simulink model "hu_flatness"  (R2017b)
settings: Solver=VariableStepAuto  StartTime=0.0  StopTime=102  RelTol=1e-9
libraries: simulink x1
(part 2 of 3)

== matlab function hu_flatness/References ==
  data: t input; references output size=18
function references = fcn(t)
%% specify your references here
g=9.81;
if t>=0 & t<2
tanalpha=-1 ; % slope
if t>=0 & t<1
   [ax_d az_d ax_d_dot az_d_dot ax_d_dot_dot az_d_dot_dot]=nest(t);
    ax_d=ax_d;                   az_d=az_d;
    ax_d_dot=ax_d_dot;           az_d_dot=az_d_dot;
    ax_d_dot_dot=ax_d_dot_dot;   az_d_dot_dot=az_d_dot_dot;
else % t>=1 & t<2
   [ax_d az_d ax_d_dot az_d_dot ax_d_dot_dot az_d_dot_dot]=nest(t-1);
  ax_d=-ax_d;                 az_d=-az_d; % invert the direction for the sake of making end velocity zero
  ax_d_dot=-ax_d_dot;         az_d_dot=-az_d_dot;
  ax_d_dot_dot=-ax_d_dot_dot; az_d_dot_dot=-az_d_dot_dot;   
end  
 r_desired=[0 0 0]'    ;              % reference's positions is not solved here
 r_desired_dot=[0 0 0]'    ;          % reference's velocities is not solved here
 r_desired_dot_dot=[ax_d 0 az_d]'   ;       % reference's accelerations
 r_desired_dot_dot_dot=[ax_d_dot 0 az_d_dot]';      % jerk
 r_desired_dot_dot_dot_dot=[ax_d_dot_dot 0 az_d_dot_dot]' ; % snap
 psi_desired=0 ;                      % reference's yaw angle
 psi_desired_dot=0 ;                  % reference's change rate of yaw angle       
 psi_desired_dot_dot=0;
 
elseif t>=2 & t<4
r_desired=[0 0 0]'    ;              % reference's positions is not solved here
r_desired_dot=[0 0 0]'    ;          % reference's velocities is not solved here
r_desired_dot_dot=[0 0 0]'   ;       % reference's accelerations
r_desired_dot_dot_dot=[0 0 0]';      % jerk
r_desired_dot_dot_dot_dot=[0 0 0]' ; % snap
if t>=2 & t<3
psi_desired=pi/4*(t-2)^2 ;                      % reference's yaw angle
psi_desired_dot=pi/2*(t-2);                  % reference's change rate of yaw angle       
psi_desired_dot_dot=pi/2; 
else % t>=3 & t<4
psi_desired=-pi/4*(t-4)^2+pi/2 ;                      % reference's yaw angle
psi_desired_dot=-pi/2*(t-4);                  % reference's change rate of yaw angle       
psi_desired_dot_dot=-pi/2; 
end 

elseif t>=4 & t<6
tanalpha=1/2;
if t>=4 & t<5
   [ax_d az_d ax_d_dot az_d_dot ax_d_dot_dot az_d_dot_dot]=nest(t-4);
    ax_d=-ax_d;                  az_d=-az_d;
    ax_d_dot=-ax_d_dot;          az_d_dot=-az_d_dot;
    ax_d_dot_dot=-ax_d_dot_dot;  az_d_dot_dot=-az_d_dot_dot;
else % t>=5 & t<6
   [ax_d az_d ax_d_dot az_d_dot ax_d_dot_dot az_d_dot_dot]=nest(t-5);
  ax_d=ax_d;                 az_d=az_d; % invert the direction for the sake of making end velocity zero
  ax_d_dot=ax_d_dot;         az_d_dot=az_d_dot;
  ax_d_dot_dot=ax_d_dot_dot; az_d_dot_dot=az_d_dot_dot;   
end  
 r_desired=[0 0 0]'    ;                    % reference's positions is not solved here
 r_desired_dot=[0 0 0]'    ;                % reference's velocities is not solved here
 r_desired_dot_dot=[ax_d 0 az_d]'   ;       % reference's accelerations
 r_desired_dot_dot_dot=[ax_d_dot 0 az_d_dot]';              % jerk
 r_desired_dot_dot_dot_dot=[ax_d_dot_dot 0 az_d_dot_dot]' ; % snap
 psi_desired=pi/2 ;                      % reference's yaw angle
 psi_desired_dot=0 ;                  % reference's change rate of yaw angle       
 psi_desired_dot_dot=0;

elseif t>=6 & t<8
r_desired=[0 0 0]'    ;              % reference's positions is not solved here
r_desired_dot=[0 0 0]'    ;          % reference's velocities is not solved here
r_desired_dot_dot=[0 0 0]'   ;       % reference's accelerations
r_desired_dot_dot_dot=[0 0 0]';      % jerk
r_desired_dot_dot_dot_dot=[0 0 0]' ; % snap
if t>=6 & t<7
psi_desired=pi/2-pi/4*(t-6)^2 ;                      % reference's yaw angle
psi_desired_dot=-pi/2*(t-6);                  % reference's change rate of yaw angle       
psi_desired_dot_dot=-pi/2; 
else % t>=7 & t<8
psi_desired=pi/4*(t-8)^2 ;                      % reference's yaw angle
psi_desired_dot=pi/2*(t-8);                  % reference's change rate of yaw angle       
psi_desired_dot_dot=pi/2; 
end

elseif t>=8 & t<10
tanalpha=-1;
if t>=8 & t<9
   [ax_d az_d ax_d_dot az_d_dot ax_d_dot_dot az_d_dot_dot]=nest(t-8);
    ax_d=ax_d;                        az_d=az_d;
    ax_d_dot=ax_d_dot;           az_d_dot=az_d_dot;
    ax_d_dot_dot=ax_d_dot_dot;   az_d_dot_dot=az_d_dot_dot;
else % t>=9 & t<10
   [ax_d az_d ax_d_dot az_d_dot ax_d_dot_dot az_d_dot_dot]=nest(t-9);
  ax_d=-ax_d;                 az_d=-az_d; % invert the direction for the sake of making end velocity zero
  ax_d_dot=-ax_d_dot;         az_d_dot=-az_d_dot;
  ax_d_dot_dot=-ax_d_dot_dot; az_d_dot_dot=-az_d_dot_dot;   
end  
 r_desired=[0 0 0]'    ;              % reference's positions is not solved here
 r_desired_dot=[0 0 0]'    ;          % reference's velocities is not solved here
 r_desired_dot_dot=[ax_d 0 az_d]'   ;       % reference's accelerations
 r_desired_dot_dot_dot=[ax_d_dot 0 az_d_dot]';      % jerk
 r_desired_dot_dot_dot_dot=[ax_d_dot_dot 0 az_d_dot_dot]' ; % snap
 psi_desired=0 ;                      % reference's yaw angle
 psi_desired_dot=0 ;                  % reference's change rate of yaw angle       
 psi_desired_dot_dot=0;

elseif t>=10 & t<12
r_desired=[0 0 0]'    ;              % reference's positions is not solved here
r_desired_dot=[0 0 0]'    ;          % reference's velocities is not solved here
r_desired_dot_dot=[0 0 0]'   ;       % reference's accelerations
r_desired_dot_dot_dot=[0 0 0]';      % jerk
r_desired_dot_dot_dot_dot=[0 0 0]' ; % snap
if t>=10 & t<11
psi_desired=pi/4*(t-10)^2 ;                      % reference's yaw angle
psi_desired_dot=pi/2*(t-10);                  % reference's change rate of yaw angle       
psi_desired_dot_dot=pi/2; 
else % t>=11 & t<12
psi_desired=-pi/4*(t-12)^2+pi/2 ;                      % reference's yaw angle
psi_desired_dot=-pi/2*(t-12);                  % reference's change rate of yaw angle       
psi_desired_dot_dot=-pi/2; 
end 

elseif t>=12 & t<14
tanalpha=2;
if t>=12 & t<13
   [ax_d az_d ax_d_dot az_d_dot ax_d_dot_dot az_d_dot_dot]=nest(t-12);
    ax_d=-ax_d;                  az_d=-az_d;
    ax_d_dot=-ax_d_dot;          az_d_dot=-az_d_dot;
    ax_d_dot_dot=-ax_d_dot_dot;  az_d_dot_dot=-az_d_dot_dot;
else % t>=13 & t<14
   [ax_d az_d ax_d_dot az_d_dot ax_d_dot_dot az_d_dot_dot]=nest(t-13);
  ax_d=ax_d;                 az_d=az_d; % invert the direction for the sake of making end velocity zero
  ax_d_dot=ax_d_dot;         az_d_dot=az_d_dot;
  ax_d_dot_dot=ax_d_dot_dot; az_d_dot_dot=az_d_dot_dot;   
end  
 r_desired=[0 0 0]'    ;                    % reference's positions is not solved here
 r_desired_dot=[0 0 0]'    ;                % reference's velocities is not solved here
 r_desired_dot_dot=[ax_d 0 az_d]'   ;       % reference's accelerations
 r_desired_dot_dot_dot=[ax_d_dot 0 az_d_dot]';              % jerk
 r_desired_dot_dot_dot_dot=[ax_d_dot_dot 0 az_d_dot_dot]' ; % snap
 psi_desired=pi/2 ;                      % reference's yaw angle
 psi_desired_dot=0 ;                  % reference's change rate of yaw angle       
 psi_desired_dot_dot=0; 
 
elseif t>=14 & t<16
r_desired=[0 0 0]'    ;              % reference's positions is not solved here
r_desired_dot=[0 0 0]'    ;          % reference's velocities is not solved here
r_desired_dot_dot=[0 0 0]'   ;       % reference's accelerations
r_desired_dot_dot_dot=[0 0 0]';      % jerk
r_desired_dot_dot_dot_dot=[0 0 0]' ; % snap
if t>=14 & t<15
psi_desired=pi/2-pi/4*(t-14)^2 ;                      % reference's yaw angle
psi_desired_dot=-pi/2*(t-14);                  % reference's change rate of yaw angle       
psi_desired_dot_dot=-pi/2; 
else % t>=15 & t<16
psi_desired=pi/4*(t-16)^2 ;                      % reference's yaw angle
psi_desired_dot=pi/2*(t-16);                  % reference's change rate of yaw angle       
psi_desired_dot_dot=pi/2; 
end

elseif t>=16 & t<18
tanalpha=5/3;
if t>=16 & t<17
   [ax_d az_d ax_d_dot az_d_dot ax_d_dot_dot az_d_dot_dot]=nest(t-16);
    ax_d=ax_d;                   az_d=az_d;
    ax_d_dot=ax_d_dot;           az_d_dot=az_d_dot;
    ax_d_dot_dot=ax_d_dot_dot;   az_d_dot_dot=az_d_dot_dot;
else % t>=17 & t<18
   [ax_d az_d ax_d_dot az_d_dot ax_d_dot_dot az_d_dot_dot]=nest(t-17);
  ax_d=-ax_d;                 az_d=-az_d; % invert the direction for the sake of making end velocity zero
  ax_d_dot=-ax_d_dot;         az_d_dot=-az_d_dot;
  ax_d_dot_dot=-ax_d_dot_dot; az_d_dot_dot=-az_d_dot_dot;   
end  
 r_desired=[0 0 0]'    ;              % reference's positions is not solved here
 r_desired_dot=[0 0 0]'    ;          % reference's velocities is not solved here
 r_desired_dot_dot=[ax_d 0 az_d]'   ;       % reference's accelerations
 r_desired_dot_dot_dot=[ax_d_dot 0 az_d_dot]';      % jerk
 r_desired_dot_dot_dot_dot=[ax_d_dot_dot 0 az_d_dot_dot]' ; % snap
 psi_desired=0 ;                      % reference's yaw angle
 psi_desired_dot=0 ;                  % reference's change rate of yaw angle       
 psi_desired_dot_dot=0;
 
elseif t>=18 & t<20
r_desired=[0 0 0]'    ;              % reference's positions is not solved here
r_desired_dot=[0 0 0]'    ;          % reference's velocities is not solved here
r_desired_dot_dot=[0 0 0]'   ;       % reference's accelerations
r_desired_dot_dot_dot=[0 0 0]';      % jerk
r_desired_dot_dot_dot_dot=[0 0 0]' ; % snap
if t>=18 & t<19
psi_desired=pi/4*(t-18)^2 ;                      % reference's yaw angle
psi_desired_dot=pi/2*(t-18);                  % reference's change rate of yaw angle       
psi_desired_dot_dot=pi/2; 
else % t>=19 & t<20
psi_desired=-pi/4*(t-20)^2+pi/2 ;                      % reference's yaw angle
psi_desired_dot=-pi/2*(t-20);                  % reference's change rate of yaw angle       
psi_desired_dot_dot=-pi/2; 
end 

elseif t>=20 & t<22
tanalpha=6 ; % slope
if t>=20 & t<21
   [ax_d az_d ax_d_dot az_d_dot ax_d_dot_dot az_d_dot_dot]=nest(t-20);
    ax_d=1/6*ax_d;                   az_d=1/6*az_d;
    ax_d_dot=1/6*ax_d_dot;           az_d_dot=1/6*az_d_dot;
    ax_d_dot_dot=1/6*ax_d_dot_dot;   az_d_dot_dot=1/6*az_d_dot_dot;
else % t>=21 & t<22
   [ax_d az_d ax_d_dot az_d_dot ax_d_dot_dot az_d_dot_dot]=nest(t-21);
  ax_d=-1/6*ax_d;                 az_d=-1/6*az_d; % invert the direction for the sake of making end velocity zero
  ax_d_dot=-1/6*ax_d_dot;         az_d_dot=-1/6*az_d_dot;
  ax_d_dot_dot=-1/6*ax_d_dot_dot; az_d_dot_dot=-1/6*az_d_dot_dot;   
end  
 r_desired=[0 0 0]'    ;              % reference's positions is not solved here
 r_desired_dot=[0 0 0]'    ;          % reference's velocities is not solved here
 r_desired_dot_dot=[ax_d 0 az_d]'   ;       % reference's accelerations
 r_desired_dot_dot_dot=[ax_d_dot 0 az_d_dot]';      % jerk
 r_desired_dot_dot_dot_dot=[ax_d_dot_dot 0 az_d_dot_dot]' ; % snap
 psi_desired=pi/2 ;                      % reference's yaw angle
 psi_desired_dot=0 ;                  % reference's change rate of yaw angle       
 psi_desired_dot_dot=0;

elseif t>=22 & t<24
r_desired=[0 0 0]'    ;              % reference's positions is not solved here
r_desired_dot=[0 0 0]'    ;          % reference's velocities is not solved here
r_desired_dot_dot=[0 0 0]'   ;       % reference's accelerations
r_desired_dot_dot_dot=[0 0 0]';      % jerk
r_desired_dot_dot_dot_dot=[0 0 0]' ; % snap
if t>=22 & t<23
psi_desired=pi/2-pi/4*(t-22)^2 ;                      % reference's yaw angle
psi_desired_dot=-pi/2*(t-22);                  % reference's change rate of yaw angle       
psi_desired_dot_dot=-pi/2; 
else % t>=23 & t<24
psi_desired=pi/4*(t-24)^2 ;                      % reference's yaw angle
psi_desired_dot=pi/2*(t-24);                  % reference's change rate of yaw angle       
psi_desired_dot_dot=pi/2; 
end

elseif t>=24 & t<26
tanalpha=0 ; % slope
if t>=24 & t<25
   [ax_d az_d ax_d_dot az_d_dot ax_d_dot_dot az_d_dot_dot]=nest(t-24);
    ax_d=4/3*ax_d;                   az_d=4/3*az_d;
    ax_d_dot=4/3*ax_d_dot;           az_d_dot=4/3*az_d_dot;
    ax_d_dot_dot=4/3*ax_d_dot_dot;   az_d_dot_dot=4/3*az_d_dot_dot;
else % t>=25 & t<26
   [ax_d az_d ax_d_dot az_d_dot ax_d_dot_dot az_d_dot_dot]=nest(t-25);
  ax_d=-4/3*ax_d;                 az_d=-4/3*az_d; % invert the direction for the sake of making end velocity zero
  ax_d_dot=-4/3*ax_d_dot;         az_d_dot=-4/3*az_d_dot;
  ax_d_dot_dot=-4/3*ax_d_dot_dot; az_d_dot_dot=-4/3*az_d_dot_dot;   
end  
 r_desired=[0 0 0]'    ;              % reference's positions is not solved here
 r_desired_dot=[0 0 0]'    ;          % reference's velocities is not solved here
 r_desired_dot_dot=[ax_d 0 az_d]'   ;       % reference's accelerations
 r_desired_dot_dot_dot=[ax_d_dot 0 az_d_dot]';      % jerk
 r_desired_dot_dot_dot_dot=[ax_d_dot_dot 0 az_d_dot_dot]' ; % snap
 psi_desired=0 ;                      % reference's yaw angle
 psi_desired_dot=0 ;                  % reference's change rate of yaw angle       
 psi_desired_dot_dot=0;
 
elseif t>=26 & t<28
r_desired=[0 0 0]'    ;              % reference's positions is not solved here
r_desired_dot=[0 0 0]'    ;          % reference's velocities is not solved here
r_desired_dot_dot=[0 0 0]'   ;       % reference's accelerations
r_desired_dot_dot_dot=[0 0 0]';      % jerk
r_desired_dot_dot_dot_dot=[0 0 0]' ; % snap
if t>=26 & t<27
psi_desired=pi/4*(t-26)^2 ;                      % reference's yaw angle
psi_desired_dot=pi/2*(t-26);                  % reference's change rate of yaw angle       
psi_desired_dot_dot=pi/2; 
else % t>=27 & t<28
psi_desired=-pi/4*(t-28)^2+pi/2 ;                      % reference's yaw angle
psi_desired_dot=-pi/2*(t-28);                  % reference's change rate of yaw angle       
psi_desired_dot_dot=-pi/2; 
end 

elseif t>=28 & t<30
tanalpha=-2;
if t>=28 & t<29
   [ax_d az_d ax_d_dot az_d_dot ax_d_dot_dot az_d_dot_dot]=nest(t-28);
    ax_d=-214/292*ax_d;                  az_d=-214/292*az_d;
    ax_d_dot=-214/292*ax_d_dot;          az_d_dot=-214/292*az_d_dot;
    ax_d_dot_dot=-214/292*ax_d_dot_dot;  az_d_dot_dot=-214/292*az_d_dot_dot;
else % t>=29 & t<30
   [ax_d az_d ax_d_dot az_d_dot ax_d_dot_dot az_d_dot_dot]=nest(t-29);
  ax_d=214/292*ax_d;                 az_d=214/292*az_d; % invert the direction for the sake of making end velocity zero
  ax_d_dot=214/292*ax_d_dot;         az_d_dot=214/292*az_d_dot;
  ax_d_dot_dot=214/292*ax_d_dot_dot; az_d_dot_dot=214/292*az_d_dot_dot;   
end  
 r_desired=[0 0 0]'    ;                    % reference's positions is not solved here
 r_desired_dot=[0 0 0]'    ;                % reference's velocities is not solved here
 r_desired_dot_dot=[ax_d 0 az_d]'   ;       % reference's accelerations
 r_desired_dot_dot_dot=[ax_d_dot 0 az_d_dot]';              % jerk
 r_desired_dot_dot_dot_dot=[ax_d_dot_dot 0 az_d_dot_dot]' ; % snap
 psi_desired=pi/2 ;                      % reference's yaw angle
 psi_desired_dot=0 ;                  % reference's change rate of yaw angle       
 psi_desired_dot_dot=0;

elseif t>=30 & t<32
r_desired=[0 0 0]'    ;              % reference's positions is not solved here
r_desired_dot=[0 0 0]'    ;          % reference's velocities is not solved here
r_desired_dot_dot=[0 0 0]'   ;       % reference's accelerations
r_desired_dot_dot_dot=[0 0 0]';      % jerk
r_desired_dot_dot_dot_dot=[0 0 0]' ; % snap
if t>=30 & t<31
psi_desired=pi/2-pi/4*(t-30)^2 ;                      % reference's yaw angle
psi_desired_dot=-pi/2*(t-30);                  % reference's change rate of yaw angle       
psi_desired_dot_dot=-pi/2; 
else % t>=31 & t<32
psi_desired=pi/4*(t-32)^2 ;                      % reference's yaw angle
psi_desired_dot=pi/2*(t-32);                  % reference's change rate of yaw angle       
psi_desired_dot_dot=pi/2; 
end

elseif t>=32 & t<34
if t>=32 & t<33
 r_desired=[0 0 0]'    ;              % reference's positions not solved
 r_desired_dot=[0 0 0]'    ;          % reference's velocities not solved
 r_desired_dot_dot=[0 0 -4/5]'   ;       % reference's accelerations
 r_desired_dot_dot_dot=[0 0 0]';      % jerk
 r_desired_dot_dot_dot_dot=[0 0 0]' ; % snap
else % t>=33 & t<34
 r_desired=[0 0 0]'    ;              % reference's positions not solved
 r_desired_dot=[0 0 0]'    ;          % reference's velocities not solved
 r_desired_dot_dot=[0 0 4/5]'   ;       % reference's accelerations
 r_desired_dot_dot_dot=[0 0 0]';      % jerk
 r_desired_dot_dot_dot_dot=[0 0 0]' ; % snap
end
 psi_desired=0 ;                      % reference's yaw angle
 psi_desired_dot=0 ;                  % reference's change rate of yaw angle       
 psi_desired_dot_dot=0;
 
elseif t>=34 & t<36
r_desired=[0 0 0]'    ;              % reference's positions is not solved here
r_desired_dot=[0 0 0]'    ;          % reference's velocities is not solved here
r_desired_dot_dot=[0 0 0]'   ;       % reference's accelerations
r_desired_dot_dot_dot=[0 0 0]';      % jerk
r_desired_dot_dot_dot_dot=[0 0 0]' ; % snap
if t>=34 & t<35
psi_desired=pi/4*(t-34)^2 ;                      % reference's yaw angle
psi_desired_dot=pi/2*(t-34);                  % reference's change rate of yaw angle       
psi_desired_dot_dot=pi/2; 
else % t>=35 & t<36
psi_desired=-pi/4*(t-36)^2+pi/2 ;                      % reference's yaw angle
psi_desired_dot=-pi/2*(t-36);                  % reference's change rate of yaw angle       
psi_desired_dot_dot=-pi/2; 
end 

elseif t>=36 & t<38
tanalpha=0 ; % slope
if t>=36 & t<37
   [ax_d az_d ax_d_dot az_d_dot ax_d_dot_dot az_d_dot_dot]=nest(t-36);
    ax_d=-1/2*ax_d;                   az_d=-1/2*az_d;
    ax_d_dot=-1/2*ax_d_dot;           az_d_dot=-1/2*az_d_dot;
    ax_d_dot_dot=-1/2*ax_d_dot_dot;   az_d_dot_dot=-1/2*az_d_dot_dot;
else % t>=37 & t<38
   [ax_d az_d ax_d_dot az_d_dot ax_d_dot_dot az_d_dot_dot]=nest(t-37);
  ax_d=1/2*ax_d;                 az_d=1/2*az_d; % invert the direction for the sake of making end velocity zero
  ax_d_dot=1/2*ax_d_dot;         az_d_dot=1/2*az_d_dot;
  ax_d_dot_dot=1/2*ax_d_dot_dot; az_d_dot_dot=1/2*az_d_dot_dot;   
end  
 r_desired=[0 0 0]'    ;              % reference's positions is not solved here
 r_desired_dot=[0 0 0]'    ;          % reference's velocities is not solved here
 r_desired_dot_dot=[ax_d 0 az_d]'   ;       % reference's accelerations
 r_desired_dot_dot_dot=[ax_d_dot 0 az_d_dot]';      % jerk
 r_desired_dot_dot_dot_dot=[ax_d_dot_dot 0 az_d_dot_dot]' ; % snap
 psi_desired=pi/2 ;                      % reference's yaw angle
 psi_desired_dot=0 ;                  % reference's change rate of yaw angle       
 psi_desired_dot_dot=0;
 
elseif t>=38 & t<40
r_desired=[0 0 0]'    ;              % reference's positions is not solved here
r_desired_dot=[0 0 0]'    ;          % reference's velocities is not solved here
r_desired_dot_dot=[0 0 0]'   ;       % reference's accelerations
r_desired_dot_dot_dot=[0 0 0]';      % jerk
r_desired_dot_dot_dot_dot=[0 0 0]' ; % snap
if t>=38 & t<39
psi_desired=pi/2-pi/4*(t-38)^2 ;                      % reference's yaw angle
psi_desired_dot=-pi/2*(t-38);                  % reference's change rate of yaw angle       
psi_desired_dot_dot=-pi/2; 
else % t>=39 & t<40
psi_desired=pi/4*(t-40)^2 ;                      % reference's yaw angle
psi_desired_dot=pi/2*(t-40);                  % reference's change rate of yaw angle       
psi_desired_dot_dot=pi/2; 
end

elseif t>=40 & t<42
if t>=40 & t<41
 r_desired=[0 0 0]'    ;              % reference's positions not solved
 r_desired_dot=[0 0 0]'    ;          % reference's velocities not solved
 r_desired_dot_dot=[0 0 -1/2]'   ;       % reference's accelerations
 r_desired_dot_dot_dot=[0 0 0]';      % jerk
 r_desired_dot_dot_dot_dot=[0 0 0]' ; % snap
else % t>=41 & t<42
 r_desired=[0 0 0]'    ;              % reference's positions not solved
 r_desired_dot=[0 0 0]'    ;          % reference's velocities not solved
 r_desired_dot_dot=[0 0 1/2]'   ;       % reference's accelerations
 r_desired_dot_dot_dot=[0 0 0]';      % jerk
 r_desired_dot_dot_dot_dot=[0 0 0]' ; % snap
end
 psi_desired=0 ;                      % reference's yaw angle
 psi_desired_dot=0 ;                  % reference's change rate of yaw angle       
 psi_desired_dot_dot=0;
 
elseif t>=42 & t<44
r_desired=[0 0 0]'    ;              % reference's positions is not solved here
r_desired_dot=[0 0 0]'    ;          % reference's velocities is not solved here
r_desired_dot_dot=[0 0 0]'   ;       % reference's accelerations
r_desired_dot_dot_dot=[0 0 0]';      % jerk
r_desired_dot_dot_dot_dot=[0 0 0]' ; % snap
if t>=42 & t<43
psi_desired=pi/4*(t-42)^2 ;                      % reference's yaw angle
psi_desired_dot=pi/2*(t-42);                  % reference's change rate of yaw angle       
psi_desired_dot_dot=pi/2; 
else % t>=43 & t<44
psi_desired=-pi/4*(t-44)^2+pi/2 ;                      % reference's yaw angle
psi_desired_dot=-pi/2*(t-44);                  % reference's change rate of yaw angle       
psi_desired_dot_dot=-pi/2; 
end 

elseif t>=44 & t<46
if t>=44 & t<45
 r_desired=[0 0 0]'    ;              % reference's positions not solved
 r_desired_dot=[0 0 0]'    ;          % reference's velocities not solved
 r_desired_dot_dot=[0 0 1/2]'   ;       % reference's accelerations
 r_desired_dot_dot_dot=[0 0 0]';      % jerk
 r_desired_dot_dot_dot_dot=[0 0 0]' ; % snap
else % t>=45 & t<46
 r_desired=[0 0 0]'    ;              % reference's positions not solved
 r_desired_dot=[0 0 0]'    ;          % reference's velocities not solved
 r_desired_dot_dot=[0 0 -1/2]'   ;       % reference's accelerations
 r_desired_dot_dot_dot=[0 0 0]';      % jerk
 r_desired_dot_dot_dot_dot=[0 0 0]' ; % snap
end
 psi_desired=pi/2 ;                      % reference's yaw angle
 psi_desired_dot=0 ;                  % reference's change rate of yaw angle       
 psi_desired_dot_dot=0;
 
elseif t>=46 & t<48
r_desired=[0 0 0]'    ;              % reference's positions is not solved here
r_desired_dot=[0 0 0]'    ;          % reference's velocities is not solved here
r_desired_dot_dot=[0 0 0]'   ;       % reference's accelerations
r_desired_dot_dot_dot=[0 0 0]';      % jerk
r_desired_dot_dot_dot_dot=[0 0 0]' ; % snap
if t>=46 & t<47
psi_desired=pi/2-pi/4*(t-46)^2 ;                      % reference's yaw angle
psi_desired_dot=-pi/2*(t-46);                  % reference's change rate of yaw angle       
psi_desired_dot_dot=-pi/2; 
else % t>=47 & t<48
psi_desired=pi/4*(t-48)^2 ;                      % reference's yaw angle
psi_desired_dot=pi/2*(t-48);                  % reference's change rate of yaw angle       
psi_desired_dot_dot=pi/2; 
end

elseif t>=48 & t<50
tanalpha=0 ; % slope
if t>=48 & t<49
   [ax_d az_d ax_d_dot az_d_dot ax_d_dot_dot az_d_dot_dot]=nest(t-48);
    ax_d=ax_d;                   az_d=az_d;
    ax_d_dot=ax_d_dot;           az_d_dot=az_d_dot;
    ax_d_dot_dot=ax_d_dot_dot;   az_d_dot_dot=az_d_dot_dot;
else % t>=49 & t<50
   [ax_d az_d ax_d_dot az_d_dot ax_d_dot_dot az_d_dot_dot]=nest(t-49);
  ax_d=-ax_d;                 az_d=-az_d; % invert the direction for the sake of making end velocity zero
  ax_d_dot=-ax_d_dot;         az_d_dot=-az_d_dot;
  ax_d_dot_dot=-ax_d_dot_dot; az_d_dot_dot=-az_d_dot_dot;   
end  
 r_desired=[0 0 0]'    ;              % reference's positions is not solved here
 r_desired_dot=[0 0 0]'    ;          % reference's velocities is not solved here
 r_desired_dot_dot=[ax_d 0 az_d]'   ;       % reference's accelerations
 r_desired_dot_dot_dot=[ax_d_dot 0 az_d_dot]';      % jerk
 r_desired_dot_dot_dot_dot=[ax_d_dot_dot 0 az_d_dot_dot]' ; % snap
 psi_desired=0 ;                      % reference's yaw angle
 psi_desired_dot=0 ;                  % reference's change rate of yaw angle       
 psi_desired_dot_dot=0;
 
elseif t>=50 & t<52
if t>=50 & t<51
 r_desired=[0 0 0]'    ;              % reference's positions not solved
 r_desired_dot=[0 0 0]'    ;          % reference's velocities not solved
 r_desired_dot_dot=[0 0 -1/2]'   ;       % reference's accelerations
 r_desired_dot_dot_dot=[0 0 0]';      % jerk
 r_desired_dot_dot_dot_dot=[0 0 0]' ; % snap
else % t>=51 & t<52
 r_desired=[0 0 0]'    ;              % reference's positions not solved
 r_desired_dot=[0 0 0]'    ;          % reference's velocities not solved
 r_desired_dot_dot=[0 0 1/2]'   ;       % reference's accelerations
 r_desired_dot_dot_dot=[0 0 0]';      % jerk
 r_desired_dot_dot_dot_dot=[0 0 0]' ; % snap
end
 psi_desired=0 ;                      % reference's yaw angle
 psi_desired_dot=0 ;                  % reference's change rate of yaw angle       
 psi_desired_dot_dot=0;
 
elseif t>=52 & t<54
r_desired=[0 0 0]'    ;              % reference's positions is not solved here
r_desired_dot=[0 0 0]'    ;          % reference's velocities is not solved here
r_desired_dot_dot=[0 0 0]'   ;       % reference's accelerations
r_desired_dot_dot_dot=[0 0 0]';      % jerk
r_desired_dot_dot_dot_dot=[0 0 0]' ; % snap
if t>=52 & t<53
psi_desired=pi/4*(t-52)^2 ;                      % reference's yaw angle
psi_desired_dot=pi/2*(t-52);                  % reference's change rate of yaw angle       
psi_desired_dot_dot=pi/2; 
else % t>=53 & t<54
psi_desired=-pi/4*(t-54)^2+pi/2 ;                      % reference's yaw angle
psi_desired_dot=-pi/2*(t-54);                  % reference's change rate of yaw angle       
psi_desired_dot_dot=-pi/2; 
end 

elseif t>=54 & t<56
tanalpha=0 ; % slope
if t>=54 & t<55
   [ax_d az_d ax_d_dot az_d_dot ax_d_dot_dot az_d_dot_dot]=nest(t-54);
    ax_d=-ax_d;                   az_d=-az_d;
    ax_d_dot=-ax_d_dot;           az_d_dot=-az_d_dot;
    ax_d_dot_dot=-ax_d_dot_dot;   az_d_dot_dot=-az_d_dot_dot;
else % t>=55 & t<56
   [ax_d az_d ax_d_dot az_d_dot ax_d_dot_dot az_d_dot_dot]=nest(t-55);
  ax_d=ax_d;                 az_d=az_d; % invert the direction for the sake of making end velocity zero
  ax_d_dot=ax_d_dot;         az_d_dot=az_d_dot;
  ax_d_dot_dot=ax_d_dot_dot; az_d_dot_dot=az_d_dot_dot;   
end  
 r_desired=[0 0 0]'    ;              % reference's positions is not solved here
 r_desired_dot=[0 0 0]'    ;          % reference's velocities is not solved here
 r_desired_dot_dot=[ax_d 0 az_d]'   ;       % reference's accelerations
 r_desired_dot_dot_dot=[ax_d_dot 0 az_d_dot]';      % jerk
 r_desired_dot_dot_dot_dot=[ax_d_dot_dot 0 az_d_dot_dot]' ; % snap
 psi_desired=pi/2 ;                      % reference's yaw angle
 psi_desired_dot=0 ;                  % reference's change rate of yaw angle       
 psi_desired_dot_dot=0;
 
elseif t>=56 & t<58
r_desired=[0 0 0]'    ;              % reference's positions is not solved here
r_desired_dot=[0 0 0]'    ;          % reference's velocities is not solved here
r_desired_dot_dot=[0 0 0]'   ;       % reference's accelerations
r_desired_dot_dot_dot=[0 0 0]';      % jerk
r_desired_dot_dot_dot_dot=[0 0 0]' ; % snap
if t>=56 & t<57
psi_desired=pi/2-pi/4*(t-56)^2 ;                      % reference's yaw angle
psi_desired_dot=-pi/2*(t-56);                  % reference's change rate of yaw angle       
psi_desired_dot_dot=-pi/2; 
else % t>=57 & t<58
psi_desired=pi/4*(t-58)^2 ;                      % reference's yaw angle
psi_desired_dot=pi/2*(t-58);                  % reference's change rate of yaw angle       
psi_desired_dot_dot=pi/2; 
end

elseif t>=58 & t<60
tanalpha=0 ; % slope
if t>=58 & t<59
   [ax_d az_d ax_d_dot az_d_dot ax_d_dot_dot az_d_dot_dot]=nest(t-58);
    ax_d=ax_d;                   az_d=az_d;
    ax_d_dot=ax_d_dot;           az_d_dot=az_d_dot;
    ax_d_dot_dot=ax_d_dot_dot;   az_d_dot_dot=az_d_dot_dot;
else % t>=59 & t<60
   [ax_d az_d ax_d_dot az_d_dot ax_d_dot_dot az_d_dot_dot]=nest(t-59);
  ax_d=-ax_d;                 az_d=-az_d; % invert the direction for the sake of making end velocity zero
  ax_d_dot=-ax_d_dot;         az_d_dot=-az_d_dot;
  ax_d_dot_dot=-ax_d_dot_dot; az_d_dot_dot=-az_d_dot_dot;   
end  
 r_desired=[0 0 0]'    ;              % reference's positions is not solved here
 r_desired_dot=[0 0 0]'    ;          % reference's velocities is not solved here
 r_desired_dot_dot=[ax_d 0 az_d]'   ;       % reference's accelerations
 r_desired_dot_dot_dot=[ax_d_dot 0 az_d_dot]';      % jerk
 r_desired_dot_dot_dot_dot=[ax_d_dot_dot 0 az_d_dot_dot]' ; % snap
 psi_desired=0 ;                      % reference's yaw angle
 psi_desired_dot=0 ;                  % reference's change rate of yaw angle       
 psi_desired_dot_dot=0;
 
elseif t>=60 & t<62
r_desired=[0 0 0]'    ;              % reference's positions is not solved here
r_desired_dot=[0 0 0]'    ;          % reference's velocities is not solved here
r_desired_dot_dot=[0 0 0]'   ;       % reference's accelerations
r_desired_dot_dot_dot=[0 0 0]';      % jerk
r_desired_dot_dot_dot_dot=[0 0 0]' ; % snap
if t>=60 & t<61
psi_desired=pi/4*(t-60)^2 ;                      % reference's yaw angle
psi_desired_dot=pi/2*(t-60);                  % reference's change rate of yaw angle       
psi_desired_dot_dot=pi/2; 
else % t>=61 & t<62
psi_desired=-pi/4*(t-62)^2+pi/2 ;                      % reference's yaw angle
psi_desired_dot=-pi/2*(t-62);                  % reference's change rate of yaw angle       
psi_desired_dot_dot=-pi/2; 
end 

elseif t>=62 & t<64
tanalpha=10 ; % slope
if t>=62 & t<63
   [ax_d az_d ax_d_dot az_d_dot ax_d_dot_dot az_d_dot_dot]=nest(t-62);
    ax_d=1311/7050*ax_d;                   az_d=1311/7050*az_d;
    ax_d_dot=1311/7050*ax_d_dot;           az_d_dot=1311/7050*az_d_dot;
    ax_d_dot_dot=1311/7050*ax_d_dot_dot;   az_d_dot_dot=1311/7050*az_d_dot_dot;
else % t>=63 & t<64
   [ax_d az_d ax_d_dot az_d_dot ax_d_dot_dot az_d_dot_dot]=nest(t-63);
  ax_d=-1311/7050*ax_d;                 az_d=-1311/7050*az_d; % invert the direction for the sake of making end velocity zero
  ax_d_dot=-1311/7050*ax_d_dot;         az_d_dot=-1311/7050*az_d_dot;
  ax_d_dot_dot=-1311/7050*ax_d_dot_dot; az_d_dot_dot=-1311/7050*az_d_dot_dot;   
end  
 r_desired=[0 0 0]'    ;                    % reference's positions is not solved here
 r_desired_dot=[0 0 0]'    ;                % reference's velocities is not solved here
 r_desired_dot_dot=[ax_d 0 az_d]'   ;       % reference's accelerations
 r_desired_dot_dot_dot=[ax_d_dot 0 az_d_dot]';      % jerk
 r_desired_dot_dot_dot_dot=[ax_d_dot_dot 0 az_d_dot_dot]' ; % snap
 psi_desired=pi/2 ;                      % reference's yaw angle
 psi_desired_dot=0 ;                  % reference's change rate of yaw angle       
 psi_desired_dot_dot=0;
 
elseif t>=64 & t<66
r_desired=[0 0 0]'    ;              % reference's positions is not solved here
r_desired_dot=[0 0 0]'    ;          % reference's velocities is not solved here
r_desired_dot_dot=[0 0 0]'   ;       % reference's accelerations
r_desired_dot_dot_dot=[0 0 0]';      % jerk
r_desired_dot_dot_dot_dot=[0 0 0]' ; % snap
if t>=64 & t<65
psi_desired=pi/2-pi/4*(t-64)^2 ;                      % reference's yaw angle
psi_desired_dot=-pi/2*(t-64);                  % reference's change rate of yaw angle       
psi_desired_dot_dot=-pi/2; 
else % t>=65 & t<66
psi_desired=pi/4*(t-66)^2 ;                      % reference's yaw angle
psi_desired_dot=pi/2*(t-66);                  % reference's change rate of yaw angle       
psi_desired_dot_dot=pi/2; 
end

elseif t>=66 & t<68
if t>=66 & t<67
 r_desired=[0 0 0]'    ;              % reference's positions not solved
 r_desired_dot=[0 0 0]'    ;          % reference's velocities not solved
 r_desired_dot_dot=[0 0 -1.5]'   ;       % reference's accelerations
 r_desired_dot_dot_dot=[0 0 0]';      % jerk
 r_desired_dot_dot_dot_dot=[0 0 0]' ; % snap
else % t>=67 & t<68
 r_desired=[0 0 0]'    ;              % reference's positions not solved
 r_desired_dot=[0 0 0]'    ;          % reference's velocities not solved
 r_desired_dot_dot=[0 0 1.5]'   ;       % reference's accelerations
 r_desired_dot_dot_dot=[0 0 0]';      % jerk
 r_desired_dot_dot_dot_dot=[0 0 0]' ; % snap
end
 psi_desired=0 ;                      % reference's yaw angle
 psi_desired_dot=0 ;                  % reference's change rate of yaw angle       
 psi_desired_dot_dot=0;
 
elseif t>=68 & t<70
r_desired=[0 0 0]'    ;              % reference's positions is not solved here
r_desired_dot=[0 0 0]'    ;          % reference's velocities is not solved here
r_desired_dot_dot=[0 0 0]'   ;       % reference's accelerations
r_desired_dot_dot_dot=[0 0 0]';      % jerk
r_desired_dot_dot_dot_dot=[0 0 0]' ; % snap
if t>=68 & t<69
psi_desired=pi/4*(t-68)^2 ;                      % reference's yaw angle
psi_desired_dot=pi/2*(t-68);                  % reference's change rate of yaw angle       
psi_desired_dot_dot=pi/2; 
else % t>=69 & t<70
psi_desired=-pi/4*(t-70)^2+pi/2 ;                      % reference's yaw angle
psi_desired_dot=-pi/2*(t-70);                  % reference's change rate of yaw angle       
psi_desired_dot_dot=-pi/2; 
end

elseif t>=70 & t<72
if t>=70 & t<71
 r_desired=[0 0 0]'    ;              % reference's positions not solved
 r_desired_dot=[0 0 0]'    ;          % reference's velocities not solved
 r_desired_dot_dot=[0 0 1.5]'   ;       % reference's accelerations
 r_desired_dot_dot_dot=[0 0 0]';      % jerk
 r_desired_dot_dot_dot_dot=[0 0 0]' ; % snap
else % t>=71 & t<72
 r_desired=[0 0 0]'    ;              % reference's positions not solved
 r_desired_dot=[0 0 0]'    ;          % reference's velocities not solved
 r_desired_dot_dot=[0 0 -1.5]'   ;       % reference's accelerations
 r_desired_dot_dot_dot=[0 0 0]';      % jerk
 r_desired_dot_dot_dot_dot=[0 0 0]' ; % snap
end
 psi_desired=pi/2 ;                      % reference's yaw angle
 psi_desired_dot=0 ;                  % reference's change rate of yaw angle       
 psi_desired_dot_dot=0;
 
elseif t>=72 & t<74
r_desired=[0 0 0]'    ;              % reference's positions is not solved here
r_desired_dot=[0 0 0]'    ;          % reference's velocities is not solved here
r_desired_dot_dot=[0 0 0]'   ;       % reference's accelerations
r_desired_dot_dot_dot=[0 0 0]';      % jerk
r_desired_dot_dot_dot_dot=[0 0 0]' ; % snap
if t>=72 & t<73
psi_desired=pi/2-pi/4*(t-72)^2 ;                      % reference's yaw angle
psi_desired_dot=-pi/2*(t-72);                  % reference's change rate of yaw angle       
psi_desired_dot_dot=-pi/2; 
else % t>=73 & t<74
psi_desired=pi/4*(t-74)^2 ;                      % reference's yaw angle
psi_desired_dot=pi/2*(t-74);                  % reference's change rate of yaw angle       
psi_desired_dot_dot=pi/2;    
end

elseif t>=74 & t<76
tanalpha=0 ; % slope
if t>=74 & t<75
   [ax_d az_d ax_d_dot az_d_dot ax_d_dot_dot az_d_dot_dot]=nest(t-74);
    ax_d=ax_d;                   az_d=az_d;
    ax_d_dot=ax_d_dot;           az_d_dot=az_d_dot;
    ax_d_dot_dot=ax_d_dot_dot;   az_d_dot_dot=az_d_dot_dot;
else % t>=75 & t<76
   [ax_d az_d ax_d_dot az_d_dot ax_d_dot_dot az_d_dot_dot]=nest(t-75);
  ax_d=-ax_d;                 az_d=-az_d; % invert the direction for the sake of making end velocity zero
  ax_d_dot=-ax_d_dot;         az_d_dot=-az_d_dot;
  ax_d_dot_dot=-ax_d_dot_dot; az_d_dot_dot=-az_d_dot_dot;   
end  
 r_desired=[0 0 0]'    ;              % reference's positions is not solved here
 r_desired_dot=[0 0 0]'    ;          % reference's velocities is not solved here
 r_desired_dot_dot=[ax_d 0 az_d]'   ;       % reference's accelerations
 r_desired_dot_dot_dot=[ax_d_dot 0 az_d_dot]';      % jerk
 r_desired_dot_dot_dot_dot=[ax_d_dot_dot 0 az_d_dot_dot]' ; % snap
 psi_desired=0 ;                      % reference's yaw angle
 psi_desired_dot=0 ;                  % reference's change rate of yaw angle       
 psi_desired_dot_dot=0;   
 
elseif t>=76 & t<78
if t>=76 & t<77
 r_desired=[0 0 0]'    ;              % reference's positions not solved
 r_desired_dot=[0 0 0]'    ;          % reference's velocities not solved
 r_desired_dot_dot=[0 0 -1.5]'   ;       % reference's accelerations
 r_desired_dot_dot_dot=[0 0 0]';      % jerk
 r_desired_dot_dot_dot_dot=[0 0 0]' ; % snap
else % t>=77 & t<78
 r_desired=[0 0 0]'    ;              % reference's positions not solved
 r_desired_dot=[0 0 0]'    ;          % reference's velocities not solved
 r_desired_dot_dot=[0 0 1.5]'   ;       % reference's accelerations
 r_desired_dot_dot_dot=[0 0 0]';      % jerk
 r_desired_dot_dot_dot_dot=[0 0 0]' ; % snap
end
 psi_desired=0 ;                      % reference's yaw angle
 psi_desired_dot=0 ;                  % reference's change rate of yaw angle       
 psi_desired_dot_dot=0;
 
elseif t>=78 & t<80
tanalpha=0 ; % slope
if t>=78 & t<79
   [ax_d az_d ax_d_dot az_d_dot ax_d_dot_dot az_d_dot_dot]=nest(t-78);
    ax_d=-1/3*ax_d;                   az_d=-1/3*az_d;
    ax_d_dot=-1/3*ax_d_dot;           az_d_dot=-1/3*az_d_dot;
    ax_d_dot_dot=-1/3*ax_d_dot_dot;   az_d_dot_dot=-1/3*az_d_dot_dot;
else % t>=79 & t<80
   [ax_d az_d ax_d_dot az_d_dot ax_d_dot_dot az_d_dot_dot]=nest(t-79);
  ax_d=1/3*ax_d;                 az_d=1/3*az_d; % invert the direction for the sake of making end velocity zero
  ax_d_dot=1/3*ax_d_dot;         az_d_dot=1/3*az_d_dot;
  ax_d_dot_dot=1/3*ax_d_dot_dot; az_d_dot_dot=1/3*az_d_dot_dot;   
end  
 r_desired=[0 0 0]'    ;              % reference's positions is not solved here
 r_desired_dot=[0 0 0]'    ;          % reference's velocities is not solved here
 r_desired_dot_dot=[ax_d 0 az_d]'   ;       % reference's accelerations
 r_desired_dot_dot_dot=[ax_d_dot 0 az_d_dot]';      % jerk
 r_desired_dot_dot_dot_dot=[ax_d_dot_dot 0 az_d_dot_dot]' ; % snap
 psi_desired=0 ;                      % reference's yaw angle
 psi_desired_dot=0 ;                  % reference's change rate of yaw angle       
 psi_desired_dot_dot=0;   
 
elseif t>=80 & t<82
r_desired=[0 0 0]'    ;              % reference's positions is not solved here
r_desired_dot=[0 0 0]'    ;          % reference's velocities is not solved here
r_desired_dot_dot=[0 0 0]'   ;       % reference's accelerations
r_desired_dot_dot_dot=[0 0 0]';      % jerk
r_desired_dot_dot_dot_dot=[0 0 0]' ; % snap
if t>=80 & t<81
psi_desired=pi/4*(t-80)^2 ;                      % reference's yaw angle
psi_desired_dot=pi/2*(t-80);                  % reference's change rate of yaw angle       
psi_desired_dot_dot=pi/2; 
else % t>=81 & t<82
psi_desired=-pi/4*(t-82)^2+pi/2 ;                      % reference's yaw angle
psi_desired_dot=-pi/2*(t-82);                  % reference's change rate of yaw angle       
psi_desired_dot_dot=-pi/2; 
end

elseif t>=82 & t<84
tanalpha=-5 ; % slope
if t>=82 & t<83
   [ax_d az_d ax_d_dot az_d_dot ax_d_dot_dot az_d_dot_dot]=nest(t-82);
    ax_d=-214/258*ax_d;                   az_d=-214/258*az_d;
    ax_d_dot=-214/258*ax_d_dot;           az_d_dot=-214/258*az_d_dot;
    ax_d_dot_dot=-214/258*ax_d_dot_dot;   az_d_dot_dot=-214/258*az_d_dot_dot;
else % t>=83 & t<84
   [ax_d az_d ax_d_dot az_d_dot ax_d_dot_dot az_d_dot_dot]=nest(t-83);
  ax_d=214/258*ax_d;                 az_d=214/258*az_d; % invert the direction for the sake of making end velocity zero
  ax_d_dot=214/258*ax_d_dot;         az_d_dot=214/258*az_d_dot;
  ax_d_dot_dot=214/258*ax_d_dot_dot; az_d_dot_dot=214/258*az_d_dot_dot;   
end  
 r_desired=[0 0 0]'    ;              % reference's positions is not solved here
 r_desired_dot=[0 0 0]'    ;          % reference's velocities is not solved here
 r_desired_dot_dot=[ax_d 0 az_d]'   ;       % reference's accelerations
 r_desired_dot_dot_dot=[ax_d_dot 0 az_d_dot]';      % jerk
 r_desired_dot_dot_dot_dot=[ax_d_dot_dot 0 az_d_dot_dot]' ; % snap
 psi_desired=pi/2 ;                      % reference's yaw angle
 psi_desired_dot=0 ;                  % reference's change rate of yaw angle       
 psi_desired_dot_dot=0; 
 
elseif t>=84 & t<86
r_desired=[0 0 0]'    ;              % reference's positions is not solved here
r_desired_dot=[0 0 0]'    ;          % reference's velocities is not solved here
r_desired_dot_dot=[0 0 0]'   ;       % reference's accelerations
r_desired_dot_dot_dot=[0 0 0]';      % jerk
r_desired_dot_dot_dot_dot=[0 0 0]' ; % snap
if t>=84 & t<85
psi_desired=pi/2-pi/4*(t-84)^2 ;                      % reference's yaw angle
psi_desired_dot=-pi/2*(t-84);                  % reference's change rate of yaw angle       
psi_desired_dot_dot=-pi/2; 
else % t>=85 & t<86
psi_desired=pi/4*(t-86)^2 ;                      % reference's yaw angle
psi_desired_dot=pi/2*(t-86);                  % reference's change rate of yaw angle       
psi_desired_dot_dot=pi/2; 
end

elseif t>=86 & t<88
tanalpha=0 ; % slope
if t>=86 & t<87
   [ax_d az_d ax_d_dot az_d_dot ax_d_dot_dot az_d_dot_dot]=nest(t-86);
    ax_d=ax_d;                   az_d=az_d;
    ax_d_dot=ax_d_dot;           az_d_dot=az_d_dot;
    ax_d_dot_dot=ax_d_dot_dot;   az_d_dot_dot=az_d_dot_dot;
else % t>=87 & t<88
   [ax_d az_d ax_d_dot az_d_dot ax_d_dot_dot az_d_dot_dot]=nest(t-87);
  ax_d=-ax_d;                 az_d=-az_d; % invert the direction for the sake of making end velocity zero
  ax_d_dot=-ax_d_dot;         az_d_dot=-az_d_dot;
  ax_d_dot_dot=-ax_d_dot_dot; az_d_dot_dot=-az_d_dot_dot;   
end  
 r_desired=[0 0 0]'    ;              % reference's positions is not solved here
 r_desired_dot=[0 0 0]'    ;          % reference's velocities is not solved here
 r_desired_dot_dot=[ax_d 0 az_d]'   ;       % reference's accelerations
 r_desired_dot_dot_dot=[ax_d_dot 0 az_d_dot]';      % jerk
 r_desired_dot_dot_dot_dot=[ax_d_dot_dot 0 az_d_dot_dot]' ; % snap
 psi_desired=0 ;                      % reference's yaw angle
 psi_desired_dot=0 ;                  % reference's change rate of yaw angle       
 psi_desired_dot_dot=0; 

elseif t>=88 & t<90
r_desired=[0 0 0]'    ;              % reference's positions is not solved here
r_desired_dot=[0 0 0]'    ;          % reference's velocities is not solved here
r_desired_dot_dot=[0 0 0]'   ;       % reference's accelerations
r_desired_dot_dot_dot=[0 0 0]';      % jerk
r_desired_dot_dot_dot_dot=[0 0 0]' ; % snap
if t>=88 & t<89
psi_desired=pi/4*(t-88)^2 ;                      % reference's yaw angle
psi_desired_dot=pi/2*(t-88);                  % reference's change rate of yaw angle       
psi_desired_dot_dot=pi/2; 
else % t>=89 & t<90
psi_desired=-pi/4*(t-90)^2+pi/2 ;                      % reference's yaw angle
psi_desired_dot=-pi/2*(t-90);                  % reference's change rate of yaw angle       
psi_desired_dot_dot=-pi/2; 
end 

elseif t>=90 & t<92
tanalpha=5/3 ; % slope
if t>=90 & t<91
   [ax_d az_d ax_d_dot az_d_dot ax_d_dot_dot az_d_dot_dot]=nest(t-90);
    ax_d=-321/351*ax_d;                   az_d=-321/351*az_d;
    ax_d_dot=-321/351*ax_d_dot;           az_d_dot=-321/351*az_d_dot;
    ax_d_dot_dot=-321/351*ax_d_dot_dot;   az_d_dot_dot=-321/351*az_d_dot_dot;
else % t>=91 & t<92
   [ax_d az_d ax_d_dot az_d_dot ax_d_dot_dot az_d_dot_dot]=nest(t-91);
  ax_d=321/351*ax_d;                 az_d=321/351*az_d; % invert the direction for the sake of making end velocity zero
  ax_d_dot=321/351*ax_d_dot;         az_d_dot=321/351*az_d_dot;
  ax_d_dot_dot=321/351*ax_d_dot_dot; az_d_dot_dot=321/351*az_d_dot_dot;   
end  
 r_desired=[0 0 0]'    ;              % reference's positions is not solved here
 r_desired_dot=[0 0 0]'    ;          % reference's velocities is not solved here
 r_desired_dot_dot=[ax_d 0 az_d]'   ;       % reference's accelerations
 r_desired_dot_dot_dot=[ax_d_dot 0 az_d_dot]';      % jerk
 r_desired_dot_dot_dot_dot=[ax_d_dot_dot 0 az_d_dot_dot]' ; % snap
 psi_desired=pi/2 ;                      % reference's yaw angle
 psi_desired_dot=0 ;                  % reference's change rate of yaw angle       
 psi_desired_dot_dot=0 ;
 
elseif t>=92 & t<94
r_desired=[0 0 0]'    ;              % reference's positions is not solved here
r_desired_dot=[0 0 0]'    ;          % reference's velocities is not solved here
r_desired_dot_dot=[0 0 0]'   ;       % reference's accelerations
r_desired_dot_dot_dot=[0 0 0]';      % jerk
r_desired_dot_dot_dot_dot=[0 0 0]' ; % snap
if t>=92 & t<93
psi_desired=pi/2-pi/4*(t-92)^2 ;                      % reference's yaw angle
psi_desired_dot=-pi/2*(t-92);                  % reference's change rate of yaw angle       
psi_desired_dot_dot=-pi/2; 
else % t>=93 & t<94
psi_desired=pi/4*(t-94)^2 ;                      % reference's yaw angle
psi_desired_dot=pi/2*(t-94);                  % reference's change rate of yaw angle       
psi_desired_dot_dot=pi/2; 
end

elseif t>=94 & t<96
tanalpha=0 ; % slope
if t>=94 & t<95
   [ax_d az_d ax_d_dot az_d_dot ax_d_dot_dot az_d_dot_dot]=nest(t-94);
    ax_d=ax_d;                   az_d=az_d;
    ax_d_dot=ax_d_dot;           az_d_dot=az_d_dot;
    ax_d_dot_dot=ax_d_dot_dot;   az_d_dot_dot=az_d_dot_dot;
else % t>=95 & t<96
   [ax_d az_d ax_d_dot az_d_dot ax_d_dot_dot az_d_dot_dot]=nest(t-95);
  ax_d=-ax_d;                 az_d=-az_d; % invert the direction for the sake of making end velocity zero
  ax_d_dot=-ax_d_dot;         az_d_dot=-az_d_dot;
  ax_d_dot_dot=-ax_d_dot_dot; az_d_dot_dot=-az_d_dot_dot;   
end  
 r_desired=[0 0 0]'    ;              % reference's positions is not solved here
 r_desired_dot=[0 0 0]'    ;          % reference's velocities is not solved here
 r_desired_dot_dot=[ax_d 0 az_d]'   ;       % reference's accelerations
 r_desired_dot_dot_dot=[ax_d_dot 0 az_d_dot]';      % jerk
 r_desired_dot_dot_dot_dot=[ax_d_dot_dot 0 az_d_dot_dot]' ; % snap
 psi_desired=0 ;                      % reference's yaw angle
 psi_desired_dot=0 ;                  % reference's change rate of yaw angle       
 psi_desired_dot_dot=0; 
 
elseif t>=96 & t<98
r_desired=[0 0 0]'    ;              % reference's positions is not solved here
r_desired_dot=[0 0 0]'    ;          % reference's velocities is not solved here
r_desired_dot_dot=[0 0 0]'   ;       % reference's accelerations
r_desired_dot_dot_dot=[0 0 0]';      % jerk
r_desired_dot_dot_dot_dot=[0 0 0]' ; % snap
if t>=96 & t<97
psi_desired=pi/4*(t-96)^2 ;                      % reference's yaw angle
psi_desired_dot=pi/2*(t-96);                  % reference's change rate of yaw angle       
psi_desired_dot_dot=pi/2; 
else % t>=97 & t<98
psi_desired=-pi/4*(t-98)^2+pi/2 ;                      % reference's yaw angle
psi_desired_dot=-pi/2*(t-98);                  % reference's change rate of yaw angle       
psi_desired_dot_dot=-pi/2; 
end 

elseif t>=98 & t<100
tanalpha=5/3 ; % slope
if t>=98 & t<99
   [ax_d az_d ax_d_dot az_d_dot ax_d_dot_dot az_d_dot_dot]=nest(t-98);
    ax_d=6/7*ax_d;                   az_d=6/7*az_d;
    ax_d_dot=6/7*ax_d_dot;           az_d_dot=6/7*az_d_dot;
    ax_d_dot_dot=6/7*ax_d_dot_dot;   az_d_dot_dot=6/7*az_d_dot_dot;
else % t>=99 & t<100
   [ax_d az_d ax_d_dot az_d_dot ax_d_dot_dot az_d_dot_dot]=nest(t-99);
  ax_d=-6/7*ax_d;                 az_d=-6/7*az_d; % invert the direction for the sake of making end velocity zero
  ax_d_dot=-6/7*ax_d_dot;         az_d_dot=-6/7*az_d_dot;
  ax_d_dot_dot=-6/7*ax_d_dot_dot; az_d_dot_dot=-6/7*az_d_dot_dot;   
end  
 r_desired=[0 0 0]'    ;              % reference's positions is not solved here
 r_desired_dot=[0 0 0]'    ;          % reference's velocities is not solved here
 r_desired_dot_dot=[ax_d 0 az_d]'   ;       % reference's accelerations
 r_desired_dot_dot_dot=[ax_d_dot 0 az_d_dot]';      % jerk
 r_desired_dot_dot_dot_dot=[ax_d_dot_dot 0 az_d_dot_dot]' ; % snap
 psi_desired=pi/2 ;                      % reference's yaw angle
 psi_desired_dot=0 ;                  % reference's change rate of yaw angle       
 psi_desired_dot_dot=0;  
 
else
r_desired=[0 0 0]'    ;              % reference's positions is not solved here
r_desired_dot=[0 0 0]'    ;          % reference's velocities is not solved here
r_desired_dot_dot=[0 0 0]'   ;       % reference's accelerations
r_desired_dot_dot_dot=[0 0 0]';      % jerk
r_desired_dot_dot_dot_dot=[0 0 0]' ; % snap
if t>=100 & t<101
psi_desired=pi/2-pi/4*(t-100)^2 ;                      % reference's yaw angle
psi_desired_dot=-pi/2*(t-100);                  % reference's change rate of yaw angle       
psi_desired_dot_dot=-pi/2; 
else % t>=101 & t<102
psi_desired=pi/4*(t-102)^2 ;                      % reference's yaw angle
psi_desired_dot=pi/2*(t-102);                  % reference's change rate of yaw angle       
psi_desired_dot_dot=pi/2; 
end
end

    
 function   [axn azn axn_dot azn_dot axn_dot_dot azn_dot_dot]=nest(tn)
        if tn>=0 & tn<1/4
        angle=pi/6*tn^2;               angle_dot=pi/3*tn;           angle_dot_dot=pi/3;
        elseif tn>=1/4 & tn<3/4
        angle=-pi/6*(tn-1/2)^2+pi/48;  angle_dot=-pi/3*(tn-1/2);    angle_dot_dot=-pi/3;
        else 
        angle=pi/6*(tn-1)^2;           angle_dot=pi/3*(tn-1);       angle_dot_dot=pi/3;
        end
     axn=g*tan(angle)/(1-tanalpha*tan(angle));
     azn=tanalpha*axn;
     axn_dot=g*(1+tan(angle)^2)*angle_dot/(1-tanalpha*tan(angle))^2;
     azn_dot=tanalpha*axn_dot;
     axn_dot_dot=g*(1+tan(angle)^2)*(2*angle_dot^2*(tan(angle)+tanalpha)+angle_dot_dot*(1-tanalpha*tan(angle)))/(1-tanalpha*tan(angle))^3;
     azn_dot_dot=tanalpha*axn_dot_dot;
  end





references=[r_desired;                 %  1-3
            r_desired_dot;             %  4-6
            r_desired_dot_dot;         %  7-9
            r_desired_dot_dot_dot;     %  10-12
            r_desired_dot_dot_dot_dot; %  13-15
            psi_desired;               %  16
            psi_desired_dot;           %  17
            psi_desired_dot_dot];      %  18
end
%% sources
%% -------- a horizontal circle with radius of 3 m-------------------------------
% r_desired=[3*cos(t) 3*sin(t) 0]'    ;             % reference's positions
% r_desired_dot=[-3*sin(t) 3*cos(t) 0]'    ;        % reference's velocities
% r_desired_dot_dot=[-3*cos(t) -3*sin(t) 0]'   ;    % reference's accelerations
% r_desired_dot_dot_dot=[3*sin(t) -3*cos(t) 0]';    % jerk
% r_desired_dot_dot_dot_dot=[3*cos(t) 3*sin(t) 0]' ;% snap
% psi_desired=0 ;                % reference's yaw angle
% psi_desired_dot=0 ;            % reference's change rate of yaw angle    
% psi_desired_dot_dot=0;
% [3 0 0,0 3 0,0 -acos(9.81/sqrt(9+9.81^2)) 0,3/sqrt(9+9.81^2) 0 0] % initial condition
%% -------- a vertiacal circle with radius of 3 m-------------------------------
% r_desired=[0 3*sin(t) -3*cos(t)]'    ;             % reference's positions
% r_desired_dot=[0 3*cos(t) 3*sin(t)]'    ;        % reference's velocities
% r_desired_dot_dot=[0 -3*sin(t) 3*cos(t)]'   ;    % reference's accelerations
% r_desired_dot_dot_dot=[0 -3*cos(t) -3*sin(t)]';    % jerk
% r_desired_dot_dot_dot_dot=[0 3*sin(t) -3*cos(t)]' ;% snap
% psi_desired=0 ;                % reference's yaw angle
% psi_desired_dot=0 ;            % reference's change rate of yaw angle    
% psi_desired_dot_dot=0;
%% ------------------a horizontal straight line--------------------------
% g=9.81;
%  if t>=0 & t<1 
%     theta_d=pi/6*t^2 ;           theta_d_dot=pi/3*t ;      theta_d_dot_dot=pi/3;
%  elseif t>=1 & t<3
%     theta_d=-pi/6*(t-2)^2+pi/3 ; theta_d_dot=-pi/3*(t-2) ; theta_d_dot_dot=-pi/3;
%  elseif t>=3 & t<4
%     theta_d=pi/6*(t-4)^2 ;       theta_d_dot=pi/3*(t-4) ;  theta_d_dot_dot=pi/3;
%  elseif t>=4 & t<5
%     theta_d=-pi/6*(t-4)^2 ;      theta_d_dot=-pi/3*(t-4) ; theta_d_dot_dot=-pi/3;
%  elseif t>=5 & t<7
%     theta_d=pi/6*(t-6)^2-pi/3 ;  theta_d_dot=pi/3*(t-6) ;  theta_d_dot_dot=pi/3;
%  else 
%     theta_d=-pi/6*(t-8)^2 ;      theta_d_dot=-pi/3*(t-8);  theta_d_dot_dot=-pi/3;
%  end
%  r_desired=[0 0 0]'    ;              % reference's positions is not solved here
%  r_desired_dot=[0 0 0]'    ;          % reference's velocities is not solved here
%  r_desired_dot_dot=[1/100*g*tan(theta_d) 0 0]'   ;       % reference's accelerations
%  r_desired_dot_dot_dot=[1/100*g*(1+tan(theta_d)^2)*theta_d_dot 0 0]';      % jerk
%  r_desired_dot_dot_dot_dot=[1/100*g*(1+tan(theta_d)^2)*(2*tan(theta_d)*theta_d_dot^2+theta_d_dot_dot) 0 0]' ; % snap
%  psi_desired=0 ;                      % reference's yaw angle
%  psi_desired_dot=0 ;                  % reference's change rate of yaw angle       
%  psi_desired_dot_dot=0;
%% ----- inclined straight line (2s)-----
% g=9.81;
% tanalpha=0 ; % slope
% if t<1
%    [ax_d az_d ax_d_dot az_d_dot ax_d_dot_dot az_d_dot_dot]=nest(t);
% else
%    [ax_d az_d ax_d_dot az_d_dot ax_d_dot_dot az_d_dot_dot]=nest(t-1);
%   ax_d=-ax_d; % invert the direction for the sake of making end velocity zero
%   az_d=-az_d;
%   ax_d_dot=-ax_d_dot;
%   az_d_dot=-az_d_dot;
%   ax_d_dot_dot=-ax_d_dot_dot;
%   az_d_dot_dot=-az_d_dot_dot;  
% end
%     function   [axn azn axn_dot azn_dot axn_dot_dot azn_dot_dot]=nest(tn)
%         if tn>=0 & tn<1/4
%         angle=8*pi/3*tn^2;               angle_dot=16*pi/3*tn;           angle_dot_dot=16*pi/3;
%         elseif tn>=1/4 & tn<3/4
%         angle=-8*pi/3*(tn-1/2)^2+pi/3;   angle_dot=-16*pi/3*(tn-1/2);    angle_dot_dot=-pi*16/3;
%         else 
%         angle=pi*8/3*(tn-1)^2;           angle_dot=pi*16/3*(tn-1);       angle_dot_dot=pi*16/3;
%         end
%      axn=g*tan(angle)/(1-tanalpha*tan(angle));
%      azn=tanalpha*axn;
%      axn_dot=g*(1+tan(angle)^2)*angle_dot/(1-tanalpha*tan(angle))^2;
%      azn_dot=tanalpha*axn_dot;
%      axn_dot_dot=g*(1+tan(angle)^2)*(2*angle_dot^2*(tan(angle)+tanalpha)+angle_dot_dot*(1-tanalpha*tan(angle)))/(1-tanalpha*tan(angle))^3;
%      azn_dot_dot=tanalpha*axn_dot_dot;
%     end
%  r_desired=[0 0 0]'    ;              % reference's positions is not solved here
%  r_desired_dot=[0 0 0]'    ;          % reference's velocities is not solved here
%  r_desired_dot_dot=[ax_d 0 az_d]'   ;       % reference's accelerations
%  r_desired_dot_dot_dot=[ax_d_dot 0 az_d_dot]';      % jerk
%  r_desired_dot_dot_dot_dot=[ax_d_dot_dot 0 az_d_dot_dot]' ; % snap
%  psi_desired=0 ;                      % reference's yaw angle
%  psi_desired_dot=0 ;                  % reference's change rate of yaw angle       
%  psi_desired_dot_dot=0;
%% ----------------inclined straight line(8s)-----------
% g=9.81;
% tanalpha=-2 ; % slope
% if t<4
%    [ax_d az_d ax_d_dot az_d_dot ax_d_dot_dot az_d_dot_dot]=nest(t);
% else
%    [ax_d az_d ax_d_dot az_d_dot ax_d_dot_dot az_d_dot_dot]=nest(t-4);
%   ax_d=-ax_d; % invert the direction for the sake of making end velocity zero
%   az_d=-az_d;
%   ax_d_dot=-ax_d_dot;
%   az_d_dot=-az_d_dot;
%   ax_d_dot_dot=-ax_d_dot_dot;
%   az_d_dot_dot=-az_d_dot_dot;  
% end
%     function   [axn azn axn_dot azn_dot axn_dot_dot azn_dot_dot]=nest(tn)
%         if tn>=0 & tn<1
%         angle=pi/6*tn^2;           angle_dot=pi/3*tn;      angle_dot_dot=pi/3;
%         elseif tn>=1 & tn<3
%         angle=-pi/6*(tn-2)^2+pi/3; angle_dot=-pi/3*(tn-2); angle_dot_dot=-pi/3;
%         else 
%         angle=pi/6*(tn-4)^2;       angle_dot=pi/3*(tn-4);  angle_dot_dot=pi/3;
%         end
%      axn=g*tan(angle)/(1-tanalpha*tan(angle));
%      azn=tanalpha*axn;
%      axn_dot=g*(1+tan(angle)^2)*angle_dot/(1-tanalpha*tan(angle))^2;
%      azn_dot=tanalpha*axn_dot;
%      axn_dot_dot=g*(1+tan(angle)^2)*(2*angle_dot^2*(tan(angle)+tanalpha)+angle_dot_dot*(1-tanalpha*tan(angle)))/(1-tanalpha*tan(angle))^3;
%      azn_dot_dot=tanalpha*axn_dot_dot;
%     end
%  r_desired=[0 0 0]'    ;              % reference's positions is not solved here
%  r_desired_dot=[0 0 0]'    ;          % reference's velocities is not solved here
%  r_desired_dot_dot=[ax_d 0 az_d]'   ;       % reference's accelerations
%  r_desired_dot_dot_dot=[ax_d_dot 0 az_d_dot]';      % jerk
%  r_desired_dot_dot_dot_dot=[ax_d_dot_dot 0 az_d_dot_dot]' ; % snap
%  psi_desired=0 ;                      % reference's yaw angle
%  psi_desired_dot=0 ;                  % reference's change rate of yaw angle       
%  psi_desired_dot_dot=0;
%% -----------a vertical straight line------------------
% if t<1
%  r_desired=[0 0 t^2]'    ;              % reference's positions 
%  r_desired_dot=[0 0 2*t]'    ;          % reference's velocities
%  r_desired_dot_dot=[0 0 2]'   ;       % reference's accelerations
%  r_desired_dot_dot_dot=[0 0 0]';      % jerk
%  r_desired_dot_dot_dot_dot=[0 0 0]' ; % snap
% else
%  r_desired=[0 0 -(t-2)^2+2]'    ;              % reference's positions 
%  r_desired_dot=[0 0 -2*(t-2)]'    ;          % reference's velocities 
%  r_desired_dot_dot=[0 0 -2]'   ;       % reference's accelerations
%  r_desired_dot_dot_dot=[0 0 0]';      % jerk
%  r_desired_dot_dot_dot_dot=[0 0 0]' ; % snap
% end
%  psi_desired=0 ;                      % reference's yaw angle
%  psi_desired_dot=0 ;                  % reference's change rate of yaw angle       
%  psi_desired_dot_dot=0;
%% --------W------------------------------------
% g=9.81;
% if t>=0 & t<8
%  if t>=0 & t<1 
%     theta_d=pi/6*t^2 ;           theta_d_dot=pi/3*t ;      theta_d_dot_dot=pi/3;
%  elseif t>=1 & t<3
%     theta_d=-pi/6*(t-2)^2+pi/3 ; theta_d_dot=-pi/3*(t-2) ; theta_d_dot_dot=-pi/3;
%  elseif t>=3 & t<4
%     theta_d=pi/6*(t-4)^2 ;       theta_d_dot=pi/3*(t-4) ;  theta_d_dot_dot=pi/3;
%  elseif t>=4 & t<5
%     theta_d=-pi/6*(t-4)^2 ;      theta_d_dot=-pi/3*(t-4) ; theta_d_dot_dot=-pi/3;
%  elseif t>=5 & t<7
%     theta_d=pi/6*(t-6)^2-pi/3 ;  theta_d_dot=pi/3*(t-6) ;  theta_d_dot_dot=pi/3;
%  else 
%     theta_d=-pi/6*(t-8)^2 ;      theta_d_dot=-pi/3*(t-8);  theta_d_dot_dot=-pi/3;
%  end
%  r_desired=[0 0 0]'    ;              % reference's positions is not solved here
%  r_desired_dot=[0 0 0]'    ;          % reference's velocities is not solved here
%  r_desired_dot_dot=[1/200*g*tan(theta_d) -sqrt(3)/200*g*tan(theta_d) 0]'   ;       % reference's accelerations
%  r_desired_dot_dot_dot=[1/200*g*(1+tan(theta_d)^2)*theta_d_dot -sqrt(3)/200*g*(1+tan(theta_d)^2)*theta_d_dot 0]';      % jerk
%  r_desired_dot_dot_dot_dot=[1/200*g*(1+tan(theta_d)^2)*(2*tan(theta_d)*theta_d_dot^2+theta_d_dot_dot) -sqrt(3)/200*g*(1+tan(theta_d)^2)*(2*tan(theta_d)*theta_d_dot^2+theta_d_dot_dot) 0]' ; % snap
%  psi_desired=-pi/3 ;                      % reference's yaw angle
%  psi_desired_dot=0 ;                  % reference's change rate of yaw angle       
%  psi_desired_dot_dot=0;
%  
% elseif t>=8 & t<10 
% r_desired=[0 0 0]'    ;              % reference's positions 
% r_desired_dot=[0 0 0]'    ;          % reference's velocities
% r_desired_dot_dot=[0 0 0]'   ;       % reference's accelerations
% r_desired_dot_dot_dot=[0 0 0]';      % jerk
% r_desired_dot_dot_dot_dot=[0 0 0]' ; % snap
% if t>=8 & t<9
% psi_desired=-pi/3+pi/3*(t-8)^2 ;                      % reference's yaw angle
% psi_desired_dot=pi*2/3*(t-8);                  % reference's change rate of yaw angle       
% psi_desired_dot_dot=pi*2/3; 
% else
% psi_desired=-pi/3*(t-10)^2+pi/3 ;                      % reference's yaw angle
% psi_desired_dot=-pi*2/3*(t-10);                  % reference's change rate of yaw angle       
% psi_desired_dot_dot=-pi*2/3; 
% end
% 
% elseif t>=10 & t<18
%   if t>=10 & t<11 
%     theta_d=pi/6*(t-10)^2 ;           theta_d_dot=pi/3*(t-10) ;      theta_d_dot_dot=pi/3;
%  elseif t>=11 & t<13
%     theta_d=-pi/6*(t-12)^2+pi/3 ; theta_d_dot=-pi/3*(t-12) ; theta_d_dot_dot=-pi/3;
%  elseif t>=13 & t<14
%     theta_d=pi/6*(t-14)^2 ;       theta_d_dot=pi/3*(t-14) ;  theta_d_dot_dot=pi/3;
%  elseif t>=14 & t<15
%     theta_d=-pi/6*(t-14)^2 ;      theta_d_dot=-pi/3*(t-14) ; theta_d_dot_dot=-pi/3;
%  elseif t>=15 & t<17
%     theta_d=pi/6*(t-16)^2-pi/3 ;  theta_d_dot=pi/3*(t-16) ;  theta_d_dot_dot=pi/3;
%  else 
%     theta_d=-pi/6*(t-18)^2 ;      theta_d_dot=-pi/3*(t-18);  theta_d_dot_dot=-pi/3;
%  end
%  r_desired=[0 0 0]'    ;              % reference's positions is not solved here
%  r_desired_dot=[0 0 0]'    ;          % reference's velocities is not solved here
%  r_desired_dot_dot=[1/200*g*tan(theta_d) sqrt(3)/200*g*tan(theta_d) 0]'   ;       % reference's accelerations
%  r_desired_dot_dot_dot=[1/200*g*(1+tan(theta_d)^2)*theta_d_dot sqrt(3)/200*g*(1+tan(theta_d)^2)*theta_d_dot 0]';      % jerk
%  r_desired_dot_dot_dot_dot=[1/200*g*(1+tan(theta_d)^2)*(2*tan(theta_d)*theta_d_dot^2+theta_d_dot_dot) sqrt(3)/200*g*(1+tan(theta_d)^2)*(2*tan(theta_d)*theta_d_dot^2+theta_d_dot_dot) 0]' ; % snap
%  psi_desired=pi/3 ;                      % reference's yaw angle
%  psi_desired_dot=0 ;                  % reference's change rate of yaw angle       
%  psi_desired_dot_dot=0;  
%  
% elseif t>=18 & t<20
% r_desired=[0 0 0]'    ;              % reference's positions 
% r_desired_dot=[0 0 0]'    ;          % reference's velocities
% r_desired_dot_dot=[0 0 0]'   ;       % reference's accelerations
% r_desired_dot_dot_dot=[0 0 0]';      % jerk
% r_desired_dot_dot_dot_dot=[0 0 0]' ; % snap
% if t>=18 & t<19
% psi_desired=pi/3-pi/3*(t-18)^2 ;                      % reference's yaw angle
% psi_desired_dot=-pi*2/3*(t-18);                  % reference's change rate of yaw angle       
% psi_desired_dot_dot=-pi*2/3; 
% else
% psi_desired=pi/3*(t-20)^2-pi/3 ;                      % reference's yaw angle
% psi_desired_dot=pi*2/3*(t-20);                  % reference's change rate of yaw angle       
% psi_desired_dot_dot=pi*2/3; 
% end
% 
% elseif t>=20 & t<28
%  if t>=20 & t<21 
%     theta_d=pi/6*(t-20)^2 ;           theta_d_dot=pi/3*(t-20) ;      theta_d_dot_dot=pi/3;
%  elseif t>=21 & t<23
%     theta_d=-pi/6*(t-22)^2+pi/3 ; theta_d_dot=-pi/3*(t-22) ; theta_d_dot_dot=-pi/3;
%  elseif t>=23 & t<24
%     theta_d=pi/6*(t-24)^2 ;       theta_d_dot=pi/3*(t-24) ;  theta_d_dot_dot=pi/3;
%  elseif t>=24 & t<25
%     theta_d=-pi/6*(t-24)^2 ;      theta_d_dot=-pi/3*(t-24) ; theta_d_dot_dot=-pi/3;
%  elseif t>=25 & t<27
%     theta_d=pi/6*(t-26)^2-pi/3 ;  theta_d_dot=pi/3*(t-26) ;  theta_d_dot_dot=pi/3;
%  else 
%     theta_d=-pi/6*(t-28)^2 ;      theta_d_dot=-pi/3*(t-28);  theta_d_dot_dot=-pi/3;
%  end
%  r_desired=[0 0 0]'    ;              % reference's positions is not solved here
%  r_desired_dot=[0 0 0]'    ;          % reference's velocities is not solved here
%  r_desired_dot_dot=[1/200*g*tan(theta_d) -sqrt(3)/200*g*tan(theta_d) 0]'   ;       % reference's accelerations
%  r_desired_dot_dot_dot=[1/200*g*(1+tan(theta_d)^2)*theta_d_dot -sqrt(3)/200*g*(1+tan(theta_d)^2)*theta_d_dot 0]';      % jerk
%  r_desired_dot_dot_dot_dot=[1/200*g*(1+tan(theta_d)^2)*(2*tan(theta_d)*theta_d_dot^2+theta_d_dot_dot) -sqrt(3)/200*g*(1+tan(theta_d)^2)*(2*tan(theta_d)*theta_d_dot^2+theta_d_dot_dot) 0]' ; % snap
%  psi_desired=-pi/3 ;                      % reference's yaw angle
%  psi_desired_dot=0 ;                      % reference's change rate of yaw angle       
%  psi_desired_dot_dot=0; 
%  
% elseif t>=28 & t<30
% r_desired=[0 0 0]'    ;              % reference's positions 
% r_desired_dot=[0 0 0]'    ;          % reference's velocities
% r_desired_dot_dot=[0 0 0]'   ;       % reference's accelerations
% r_desired_dot_dot_dot=[0 0 0]';      % jerk
% r_desired_dot_dot_dot_dot=[0 0 0]' ; % snap
% if t>=28 & t<29
% psi_desired=-pi/3+pi/3*(t-28)^2 ;                      % reference's yaw angle
% psi_desired_dot=pi*2/3*(t-28);                  % reference's change rate of yaw angle       
% psi_desired_dot_dot=pi*2/3; 
% else
% psi_desired=-pi/3*(t-30)^2+pi/3 ;                      % reference's yaw angle
% psi_desired_dot=-pi*2/3*(t-30);                  % reference's change rate of yaw angle       
% psi_desired_dot_dot=-pi*2/3; 
% end
% 
% else
% if t>=30 & t<31 
%     theta_d=pi/6*(t-30)^2 ;           theta_d_dot=pi/3*(t-30) ;      theta_d_dot_dot=pi/3;
%  elseif t>=31 & t<33
%     theta_d=-pi/6*(t-32)^2+pi/3 ; theta_d_dot=-pi/3*(t-32) ; theta_d_dot_dot=-pi/3;
%  elseif t>=33 & t<34
%     theta_d=pi/6*(t-34)^2 ;       theta_d_dot=pi/3*(t-34) ;  theta_d_dot_dot=pi/3;
%  elseif t>=34 & t<35
%     theta_d=-pi/6*(t-34)^2 ;      theta_d_dot=-pi/3*(t-34) ; theta_d_dot_dot=-pi/3;
%  elseif t>=35 & t<37
%     theta_d=pi/6*(t-36)^2-pi/3 ;  theta_d_dot=pi/3*(t-36) ;  theta_d_dot_dot=pi/3;
%  else 
%     theta_d=-pi/6*(t-38)^2 ;      theta_d_dot=-pi/3*(t-38);  theta_d_dot_dot=-pi/3;
%  end
%  r_desired=[0 0 0]'    ;              % reference's positions is not solved here
%  r_desired_dot=[0 0 0]'    ;          % reference's velocities is not solved here
%  r_desired_dot_dot=[1/200*g*tan(theta_d) sqrt(3)/200*g*tan(theta_d) 0]'   ;       % reference's accelerations
%  r_desired_dot_dot_dot=[1/200*g*(1+tan(theta_d)^2)*theta_d_dot sqrt(3)/200*g*(1+tan(theta_d)^2)*theta_d_dot 0]';      % jerk
%  r_desired_dot_dot_dot_dot=[1/200*g*(1+tan(theta_d)^2)*(2*tan(theta_d)*theta_d_dot^2+theta_d_dot_dot) sqrt(3)/200*g*(1+tan(theta_d)^2)*(2*tan(theta_d)*theta_d_dot^2+theta_d_dot_dot) 0]' ; % snap
%  psi_desired=pi/3 ;                      % reference's yaw angle
%  psi_desired_dot=0 ;                  % reference's change rate of yaw angle       
%  psi_desired_dot_dot=0;  
%
% end
%% ------------xi hu da xue---------
% g=9.81;
% if t>=0 & t<8
%  if t>=0 & t<1 
%     theta_d=pi/6*t^2 ;           theta_d_dot=pi/3*t ;      theta_d_dot_dot=pi/3;
%  elseif t>=1 & t<3
%     theta_d=-pi/6*(t-2)^2+pi/3 ; theta_d_dot=-pi/3*(t-2) ; theta_d_dot_dot=-pi/3;
%  elseif t>=3 & t<4
%     theta_d=pi/6*(t-4)^2 ;       theta_d_dot=pi/3*(t-4) ;  theta_d_dot_dot=pi/3;
%  elseif t>=4 & t<5
%     theta_d=-pi/6*(t-4)^2 ;      theta_d_dot=-pi/3*(t-4) ; theta_d_dot_dot=-pi/3;
%  elseif t>=5 & t<7
%     theta_d=pi/6*(t-6)^2-pi/3 ;  theta_d_dot=pi/3*(t-6) ;  theta_d_dot_dot=pi/3;
%  else % t>=7 & t<8
%     theta_d=-pi/6*(t-8)^2 ;      theta_d_dot=-pi/3*(t-8);  theta_d_dot_dot=-pi/3;
%  end
%  r_desired=[0 0 0]'    ;              % reference's positions is not solved here
%  r_desired_dot=[0 0 0]'    ;          % reference's velocities is not solved here
%  r_desired_dot_dot=[1/100*g*tan(theta_d) 0 0]'   ;       % reference's accelerations
%  r_desired_dot_dot_dot=[1/100*g*(1+tan(theta_d)^2)*theta_d_dot 0 0]';      % jerk
%  r_desired_dot_dot_dot_dot=[1/100*g*(1+tan(theta_d)^2)*(2*tan(theta_d)*theta_d_dot^2+theta_d_dot_dot) 0 0]' ; % snap
%  psi_desired=0 ;                      % reference's yaw angle
%  psi_desired_dot=0 ;                  % reference's change rate of yaw angle       
%  psi_desired_dot_dot=0;
%  
% elseif t>=8 & t<10
% r_desired=[0 0 0]'    ;              % reference's positions is not solved here
% r_desired_dot=[0 0 0]'    ;          % reference's velocities is not solved here
% r_desired_dot_dot=[0 0 0]'   ;       % reference's accelerations
% r_desired_dot_dot_dot=[0 0 0]';      % jerk
% r_desired_dot_dot_dot_dot=[0 0 0]' ; % snap
% if t>=8 & t<9
% psi_desired=pi/4*(t-8)^2 ;                      % reference's yaw angle
% psi_desired_dot=pi/2*(t-8);                  % reference's change rate of yaw angle       
% psi_desired_dot_dot=pi/2; 
% else % t>=9 & t<10
% psi_desired=-pi/4*(t-10)^2+pi/2 ;                      % reference's yaw angle
% psi_desired_dot=-pi/2*(t-10);                  % reference's change rate of yaw angle       
% psi_desired_dot_dot=-pi/2; 
% end
% 
% elseif t>=10 & t<12
% if t>=10 & t<11
%  r_desired=[0 0 -1/4*(t-10)^2]'    ;              % reference's positions 
%  r_desired_dot=[0 0 -1/2*(t-8)]'    ;          % reference's velocities
%  r_desired_dot_dot=[0 0 -1/2]'   ;       % reference's accelerations
%  r_desired_dot_dot_dot=[0 0 0]';      % jerk
%  r_desired_dot_dot_dot_dot=[0 0 0]' ; % snap
% else % t>=11 & t<12
%  r_desired=[0 0 1/4*(t-12)^2+1/2]'    ;              % reference's positions 
%  r_desired_dot=[0 0 1/2*(t-12)]'    ;          % reference's velocities 
%  r_desired_dot_dot=[0 0 1/2]'   ;       % reference's accelerations
%  r_desired_dot_dot_dot=[0 0 0]';      % jerk
%  r_desired_dot_dot_dot_dot=[0 0 0]' ; % snap
% end
%  psi_desired=pi/2;                      % reference's yaw angle
%  psi_desired_dot=0 ;                  % reference's change rate of yaw angle       
%  psi_desired_dot_dot=0;
%  
% elseif t>=12 & t<20
% if t>=12 & t<13 
%     phi_d=-pi/6*(t-12)^2 ;           phi_d_dot=-pi/3*(t-12) ;      phi_d_dot_dot=-pi/3;
%  elseif t>=13 & t<15
%     phi_d=pi/6*(t-14)^2-pi/3 ;       phi_d_dot=pi/3*(t-14) ;       phi_d_dot_dot=pi/3;
%  elseif t>=15 & t<16
%     phi_d=-pi/6*(t-16)^2 ;           phi_d_dot=-pi/3*(t-16) ;      phi_d_dot_dot=-pi/3;
%  elseif t>=16 & t<17
%     phi_d=pi/6*(t-16)^2 ;            phi_d_dot=pi/3*(t-16) ;       phi_d_dot_dot=pi/3;
%  elseif t>=17 & t<19
%     phi_d=-pi/6*(t-18)^2+pi/3 ;      phi_d_dot=-pi/3*(t-18) ;      phi_d_dot_dot=-pi/3;
%  else % t>=19 & t<20
%     phi_d=pi/6*(t-20)^2 ;            phi_d_dot=pi/3*(t-20);        phi_d_dot_dot=pi/3;
% end
%  r_desired=[0 0 0]'    ;              % reference's positions is not solved here
%  r_desired_dot=[0 0 0]'    ;          % reference's velocities is not solved here
%  r_desired_dot_dot=[1/100*g*tan(phi_d) 0 0]'   ;       % reference's accelerations
%  r_desired_dot_dot_dot=[1/100*g*(1+tan(phi_d)^2)*phi_d_dot 0 0]';      % jerk
%  r_desired_dot_dot_dot_dot=[1/100*g*(1+tan(phi_d)^2)*(2*tan(phi_d)*phi_d_dot^2+phi_d_dot_dot) 0 0]' ; % snap
%  psi_desired=pi/2 ;                      % reference's yaw angle
%  psi_desired_dot=0 ;                  % reference's change rate of yaw angle       
%  psi_desired_dot_dot=0;
%  
% elseif t>=20 & t<22
% r_desired=[0 0 0]'    ;              % reference's positions is not solved here
% r_desired_dot=[0 0 0]'    ;          % reference's velocities is not solved here
% r_desired_dot_dot=[0 0 0]'   ;       % reference's accelerations
% r_desired_dot_dot_dot=[0 0 0]';      % jerk
% r_desired_dot_dot_dot_dot=[0 0 0]' ; % snap
% if t>=20 & t<21
% psi_desired=pi/2-pi/4*(t-20)^2 ;                      % reference's yaw angle
% psi_desired_dot=-pi/2*(t-20);                  % reference's change rate of yaw angle       
% psi_desired_dot_dot=-pi/2; 
% else % t>=21 & t<22
% psi_desired=pi/4*(t-22)^2 ;                      % reference's yaw angle
% psi_desired_dot=pi/2*(t-22);                  % reference's change rate of yaw angle       
% psi_desired_dot_dot=pi/2; 
% end
% 
% else
% if t>=22 & t<23
%  r_desired=[0 0 -1/2*(t-22)^2-1/2]'    ;              % reference's positions 
%  r_desired_dot=[0 0 -(t-22)]'    ;          % reference's velocities
%  r_desired_dot_dot=[0 0 -1]'   ;       % reference's accelerations
%  r_desired_dot_dot_dot=[0 0 0]';      % jerk
%  r_desired_dot_dot_dot_dot=[0 0 0]' ; % snap
% else % t>=23 & t<24
%  r_desired=[0 0 1/2*(t-24)^2-3/2]'    ;              % reference's positions 
%  r_desired_dot=[0 0 (t-24)]'    ;          % reference's velocities 
%  r_desired_dot_dot=[0 0 1]'   ;       % reference's accelerations
%  r_desired_dot_dot_dot=[0 0 0]';      % jerk
%  r_desired_dot_dot_dot_dot=[0 0 0]' ; % snap
% end
%  psi_desired=0 ;                      % reference's yaw angle
%  psi_desired_dot=0 ;                  % reference's change rate of yaw angle       
%  psi_desired_dot_dot=0;
% 
% end
